simulink model "controladorTemp2015"  (R2015a)
settings: Solver=ode45  SolverMode=SingleTasking  StartTime=0.0  StopTime=10.0  RelTol=1e-3
undefined symbols (not defined in the file or in its folder): Cd, gama, phi
libraries: dspsrcs4 x2, simulink x1
settings Model: CovMetricSettings=dwe  CovHtmlReporting=off  covSaveCumulativeToWorkspaceVar=off  CovSaveSingleToWorkspaceVar=off  CovExternalEMLEnable=on  Creator=Raposo  LastModifiedBy=Tiago
settings DataIOCC: LimitDataPoints=off  SaveFormat=Dataset
settings DebuggingCC: SFUnexpectedBacktrackingDiag=error  SFNoUnconditionalDefaultTransitionDiag=error
settings HardwareCC: ProdBitPerPointer=64  ProdLargestAtomicFloat=Float  ProdIntDivRoundTo=Zero  ProdEndianess=LittleEndian  ProdHWDeviceType=Specified
settings ModelReferenceCC: PropagateSignalLabelsOutOfModel=on
settings GRTTargetCC: TargetLangStandard=C99 (ISO)  GeneratePreprocessorConditionals=Use local settings

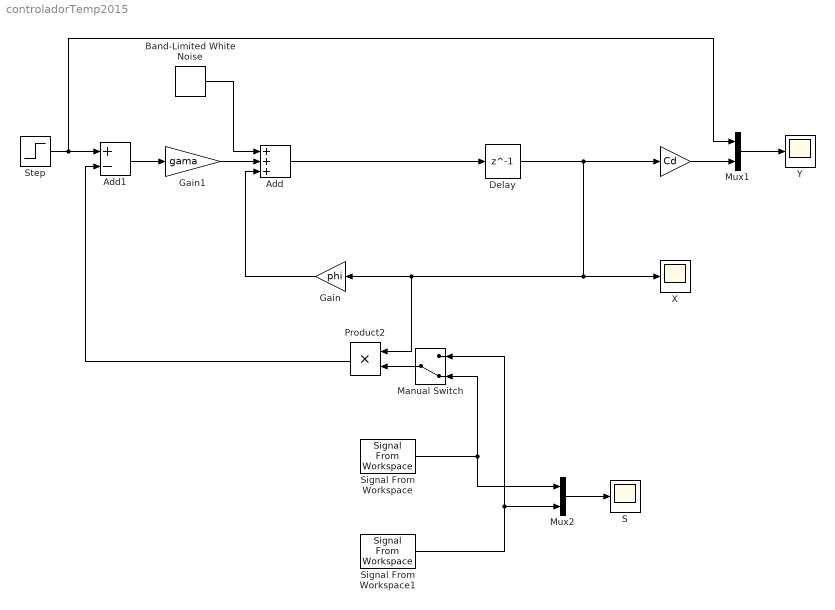
== system controladorTemp2015 ==
  " " : Gain  Gain=Cd
  Add : Sum  Inputs=+++
  Add1 : Sum  Inputs=+-
  Band-Limited White Noise : simulink/Sources/Band-Limited White Noise  Cov=[0.001]  Ts=0.1  seed=[23341]
  Delay : Delay  DelayLength=1  InitialCondition=0
  Gain : Gain  Gain=phi
  Gain1 : Gain  Gain=gama
  Manual Switch : ManualSwitch  CurrentSetting=0
  Mux1 : Mux  Inputs=2
  Mux2 : Mux  Inputs=2
  Product2 : Product
  S : Scope
      settings: TimeRange=auto  ShowLegends=on  MaxDataPoints=5000  SaveToWorkspace=off  SaveName=ScopeData3  YMin=-2.0827  YMax=4.85962  SampleTime=-1
  Signal From Workspace : dspsrcs4/Signal From Workspace  X=l  Ts=1  nsamps=1  OutputAfterFinalValue=Setting to zero  ignoreOrWarnInputAndFrameLengths=off
  Signal From Workspace1 : dspsrcs4/Signal From Workspace  X=H  Ts=1  nsamps=1  OutputAfterFinalValue=Setting to zero  ignoreOrWarnInputAndFrameLengths=off
  Step : Step  SampleTime=0
  X : Scope
      settings: TimeRange=auto  ShowLegends=on  MaxDataPoints=5000  SaveToWorkspace=off  SaveName=ScopeData  YMin=-2.0827  YMax=4.85962  SampleTime=-1
  Y : Scope
      settings: TimeRange=auto  ShowLegends=on  MaxDataPoints=5000  SaveToWorkspace=off  SaveName=ScopeData2  YMin=-2.0827  YMax=4.85962  SampleTime=-1
  wires:
  Band-Limited White Noise/1 -> Add/1
  Gain1/1 -> Add/2
  Add/1 -> Delay/1
  Gain/1 -> Add/3
  Delay/1 -> " "/1, X/1, Product2/1, Gain/1
  Signal From Workspace/1 -> Mux2/1, Manual Switch/2
  Signal From Workspace1/1 -> Mux2/2, Manual Switch/1
  Manual Switch/1 -> Product2/2
  Add1/1 -> Gain1/1
  Step/1 -> Mux1/1, Add1/1
  Product2/1 -> Add1/2
  Mux1/1 -> Y/1
  " "/1 -> Mux1/2
  Mux2/1 -> S/1
